simulink model "car"  (Simulink 8.0)
settings: Solver=ode15s  StartTime=0.0  StopTime=60  RelTol=1e-3
values from neighbouring files (symbols this model uses):
  i_f = r_back_sproket/r_front_sproket    (= 3.86486486486)    [meas_const.m]
  x = block.InputPort(1).Data    [parameterlookup.m]
undefined symbols (not defined in the file or in its folder): A_a, b, b_f, b_t, brake_gain, Bx, c_c, c_d, c_p, c_r, c_w, chaindrive, Cx, Dx, Ex, g, gearInertia, gearNumber, gearRatio, init_d, init_T, J_e, J_w, k, k_c, k_d, k_p, mass, N_idle, N_max, r_b, r_f, r_w, Rho_a, S, slope, T_max, tau_d, tau_e, x_dot
undefined symbols (not defined in the file): IdleControllerI, IdleControllerP, init_e, init_f, J_f, position
libraries: simulink x4
settings Model: Creator=erihe433  LastModifiedBy=johka546  ExtModeAutoUpdateStatusClock=off
settings DataIOCC: LimitDataPoints=off  SignalLoggingSaveFormat=ModelDataLogs  SaveOutput=off  SignalLogging=off  SignalLoggingName=sigsOut
settings OptimizationCC: InitFltsAndDblsToZero=on
settings DebuggingCC: SaveWithParameterizedLinksMsg=none  SignalResolutionControl=TryResolveAllWithWarning  SolverPrmCheckMsg=none  MultiTaskDSMMsg=warning  MultiTaskCondExecSysMsg=none  FcnCallInpInsideContextMsg=UseLocalSettings  StrictBusMsg=Warning
settings HardwareCC: TargetUnknown=on
settings RTWCC: IncludeERTFirstTime=on
settings GRTTargetCC: TargetFcnLib=ansi_tfl_tmw.mat  CombineOutputUpdateFcns=off  GRTInterface=on

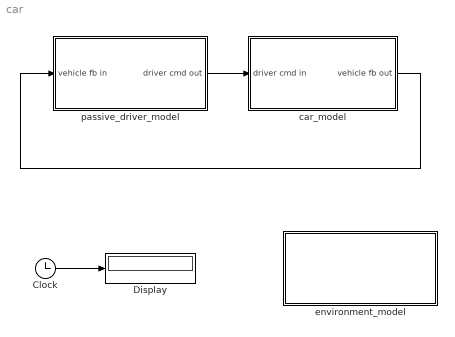
== system car ==
  Clock : Clock
  Display : Display
  car_model : Subsystem
  environment_model : Subsystem  AncestorBlock=capsim_lib/Environment/environment_model_jofr1  mask{Tamb=0, Pamb=0, pos=position, slope=slope}
      mask prompts: Tamb "Ambient Temperature [K]"; Pamb "Ambient Pressure [Pa]"; pos "positionvector in slope map [m]"; slope "slopevector in slope map [rad]"
      mask help: Environment settings
  passive_driver_model : Subsystem  AncestorBlock=capsim_lib/Driver/driver_model_template
      mask help: Driver model
  wires:
  car_model/1(vehicle fb out) -> passive_driver_model/1(vehicle fb in)
  passive_driver_model/1(driver cmd out) -> car_model/1(driver cmd in)
  Clock/1 -> Display/1

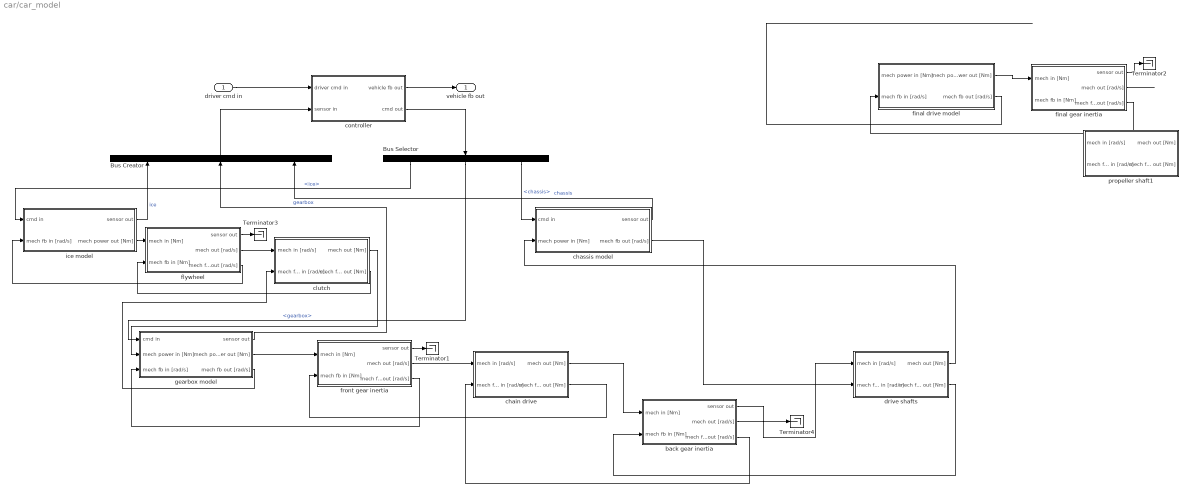
== system car/car_model ==
  driver cmd in : Inport
  Bus Creator : BusCreator  Inputs=3
  Bus Selector : BusSelector  OutputSignals=ice,gearbox,chassis
  Terminator{1..4} (4 alike) : Terminator
  back gear inertia : Subsystem  AncestorBlock=capsim_lib/Inertia/inertia_simple1_std  mask{mass=0, inertia=0, speedinit=init_f, angleinit=0}
      mask prompts: mass "Component mass [kg]"; inertia "Inertia [kg*m2]"; speedinit "Initial speed [rad/s]"; angleinit "Initial angle [rad]"
      mask help: Inertia
      mask Display: plot(-140,0,250,100,[40,40,80,80,40],[90,10,10,90,90],[80,40],[50,50],[80,40],[60,60],[80,40],[70,70],[80,40],[80,80],[80,40,40],[65,65,65],[80,40,40],[85,85,85],[80,40],[82,82],[80,40,40],[87,87,87],[80,40],[73,73],[80,40],[76,76],[80,40],[39,39],[80,40],[30,30],[80,40,40],[20,20,20],[80,40],[35,35],[80,40],[15,15],[80,40],[12,12],[80,40],[17,17],[80,40],[26,26],[80,40],[23,23],[40,10,10,40],[44,44,57,57])
  chain drive : Subsystem  AncestorBlock=capsim_lib/MechConverter/mechconverter_simple1_std  mask{mass=0, inertia=0, k_p=k_p, c_p=c_p}
      mask prompts: mass "Component mass [kg]"; inertia "Inertia [kg*m2]"; k_p "stiffness [Nm/rad]"; c_p "damping [Nms/rad]"
      mask help: Inertia
  chassis model : Subsystem  AncestorBlock=capsim_lib/Chassis/chassis_model_template
  clutch : Subsystem  AncestorBlock=capsim_lib/MechConverter/mechconverter_simple1_std  mask{mass=0, inertia=0, k_c=k_c, c_c=c_c}
      mask prompts: mass "Component mass [kg]"; inertia "Inertia [kg*m2]"; k_c "stiffness [Nm/rad]"; c_c "damping [Nms/rad]"
      mask help: Inertia
  controller : Subsystem  AncestorBlock=capsim_lib/Controller/controller_template
  drive shafts : Subsystem  AncestorBlock=capsim_lib/MechConverter/mechconverter_simple1_std  mask{mass=0, inertia=0, k_d=k_d, c_d=c_d}
      mask prompts: mass "Component mass [kg]"; inertia "Inertia [kg*m2]"; k_d "stiffness [Nm/rad]"; c_d "damping [Nms/rad]"
      mask help: Inertia
  final drive model : Subsystem  AncestorBlock=capsim_lib/Gearbox/gearbox_template
  final gear inertia : Subsystem  AncestorBlock=capsim_lib/Inertia/inertia_simple1_std  mask{mass=0, inertia=0, speedinit=init_f, angleinit=0}
      mask prompts: mass "Component mass [kg]"; inertia "Inertia [kg*m2]"; speedinit "Initial speed [rad/s]"; angleinit "Initial angle [rad]"
      mask help: Inertia
      mask Display: plot(-140,0,250,100,[40,40,80,80,40],[90,10,10,90,90],[80,40],[50,50],[80,40],[60,60],[80,40],[70,70],[80,40],[80,80],[80,40,40],[65,65,65],[80,40,40],[85,85,85],[80,40],[82,82],[80,40,40],[87,87,87],[80,40],[73,73],[80,40],[76,76],[80,40],[39,39],[80,40],[30,30],[80,40,40],[20,20,20],[80,40],[35,35],[80,40],[15,15],[80,40],[12,12],[80,40],[17,17],[80,40],[26,26],[80,40],[23,23],[40,10,10,40],[44,44,57,57])
  flywheel : Subsystem  AncestorBlock=capsim_lib/Inertia/inertia_simple1_std  mask{mass=0, inertia=0, speedinit=init_e, angleinit=0}
      mask prompts: mass "Component mass [kg]"; inertia "Inertia [kg*m2]"; speedinit "Initial speed [rad/s]"; angleinit "Initial angle [rad]"
      mask help: Inertia
      mask Display: plot(-140,0,250,100,[40,40,80,80,40],[90,10,10,90,90],[80,40],[50,50],[80,40],[60,60],[80,40],[70,70],[80,40],[80,80],[80,40,40],[65,65,65],[80,40,40],[85,85,85],[80,40],[82,82],[80,40,40],[87,87,87],[80,40],[73,73],[80,40],[76,76],[80,40],[39,39],[80,40],[30,30],[80,40,40],[20,20,20],[80,40],[35,35],[80,40],[15,15],[80,40],[12,12],[80,40],[17,17],[80,40],[26,26],[80,40],[23,23],[40,10,10,40],[44,44,57,57])
  front gear inertia : Subsystem  AncestorBlock=capsim_lib/Inertia/inertia_simple1_std  mask{mass=0, inertia=0, speedinit=init_f, angleinit=0}
      mask prompts: mass "Component mass [kg]"; inertia "Inertia [kg*m2]"; speedinit "Initial speed [rad/s]"; angleinit "Initial angle [rad]"
      mask help: Inertia
      mask Display: plot(-140,0,250,100,[40,40,80,80,40],[90,10,10,90,90],[80,40],[50,50],[80,40],[60,60],[80,40],[70,70],[80,40],[80,80],[80,40,40],[65,65,65],[80,40,40],[85,85,85],[80,40],[82,82],[80,40,40],[87,87,87],[80,40],[73,73],[80,40],[76,76],[80,40],[39,39],[80,40],[30,30],[80,40,40],[20,20,20],[80,40],[35,35],[80,40],[15,15],[80,40],[12,12],[80,40],[17,17],[80,40],[26,26],[80,40],[23,23],[40,10,10,40],[44,44,57,57])
  gearbox model : Subsystem  AncestorBlock=capsim_lib/Gearbox/gearbox_template
  ice model : Subsystem
  propeller shaft1 : Subsystem  AncestorBlock=capsim_lib/MechConverter/mechconverter_simple1_std  mask{mass=0, inertia=0, k_p=k_p, c_p=c_p}
      mask prompts: mass "Component mass [kg]"; inertia "Inertia [kg*m2]"; k_p "stiffness [Nm/rad]"; c_p "damping [Nms/rad]"
      mask help: Inertia
  vehicle fb out : Outport
  wires:
  controller/1(vehicle fb out) -> vehicle fb out/1
  driver cmd in/1 -> controller/1(driver cmd in)
  controller/2(cmd out) -> Bus Selector/1
  Bus Creator/1 -> controller/2(sensor in)
  Bus Selector/1 -> ice model/1(cmd in)  "<ice>"
  Bus Selector/3 -> chassis model/1(cmd in)  "<chassis>"
  chassis model/1(sensor out) -> Bus Creator/3  "chassis"
  ice model/2(mech power out [Nm]) -> flywheel/1(mech in [Nm])
  flywheel/3(mech fb out [rad/s]) -> ice model/2(mech fb in [rad/s])
  flywheel/2(mech out [rad/s]) -> clutch/1(mech in [rad/s])
  clutch/2(mech fb out [Nm]) -> flywheel/2(mech fb in [Nm])
  clutch/1(mech out [Nm]) -> gearbox model/2(mech power in [Nm])
  gearbox model/2(mech power out [Nm]) -> front gear inertia/1(mech in [Nm])
  gearbox model/3(mech fb out [rad/s]) -> clutch/2(mech fb in [rad/s])
  chain drive/2(mech fb out [Nm]) -> front gear inertia/2(mech fb in [Nm])
  chain drive/1(mech out [Nm]) -> back gear inertia/1(mech in [Nm])
  drive shafts/2(mech fb out [Nm]) -> back gear inertia/2(mech fb in [Nm])
  ? -> final drive model/1(mech power in [Nm])
  final drive model/2(mech fb out [rad/s]) -> ?
  final drive model/1(mech power out [Nm]) -> final gear inertia/1(mech in [Nm])
  final gear inertia/2(mech out [rad/s]) -> ?
  final gear inertia/3(mech fb out [rad/s]) -> final drive model/2(mech fb in [rad/s])
  drive shafts/1(mech out [Nm]) -> chassis model/2(mech power in [Nm])
  ? -> final gear inertia/2(mech fb in [Nm])
  chassis model/2(mech fb out [rad/s]) -> drive shafts/2(mech fb in [rad/s])
  ice model/1(sensor out) -> Bus Creator/1  "ice"
  flywheel/1(sensor out) -> Terminator3/1
  gearbox model/1(sensor out) -> Bus Creator/2  "gearbox"
  final gear inertia/1(sensor out) -> Terminator2/1
  Bus Selector/2 -> gearbox model/1(cmd in)  "<gearbox>"
  front gear inertia/2(mech out [rad/s]) -> chain drive/1(mech in [rad/s])
  front gear inertia/3(mech fb out [rad/s]) -> gearbox model/3(mech fb in [rad/s])
  front gear inertia/1(sensor out) -> Terminator1/1
  back gear inertia/3(mech fb out [rad/s]) -> chain drive/2(mech fb in [rad/s])
  back gear inertia/2(mech out [rad/s]) -> drive shafts/1(mech in [rad/s])
  back gear inertia/1(sensor out) -> Terminator4/1

== system car/environment_model ==
  Compare To Constant : simulink/Logic and Bit Operations/Compare To Constant  relop=<  const=1  OutDataTypeStr=uint8  ZeroCross=off
  Compare To Constant1 : simulink/Logic and Bit Operations/Compare To Constant  relop=<  const=1  OutDataTypeStr=uint8  ZeroCross=off
  Constant2 : Constant  Value=pos(end)
  Integrator : Integrator
  Logical Operator : Logic  Operator=OR  Inputs=3  AllPortsSameDT=off  OutDataTypeStr=boolean
  Relational Operator : RelationalOperator
  Stop Simulation1 : Stop
  To Workspace2 : ToWorkspace  VariableName=environmentout  SampleTime=-1
  slope as function of the distance : Lookup  InputValues=pos  Table=slope  LookUpMeth=Interpolation-Use End Values  SaturateOnIntegerOverflow=on
  tag scope: slope=global
  wires:
  [speed] -> Integrator/1, Compare To Constant/1
  Integrator/1 -> slope as function of the distance/1, Relational Operator/1  "distance"
  slope as function of the distance/1 -> [slope], To Workspace2/1
  Constant2/1 -> Relational Operator/2
  Logical Operator/1 -> Stop Simulation1/1
  Relational Operator/1 -> Logical Operator/1
  Compare To Constant/1 -> Logical Operator/2
  [wheelspeed] -> Compare To Constant1/1
  Compare To Constant1/1 -> Logical Operator/3

== system car/passive_driver_model ==
  vehicle fb in : Inport
  Bus Creator : BusCreator  Inputs=1
  Bus Selector : BusSelector  OutputSignals=velocity [m/s]
  From Workspace2 : FromWorkspace  VariableName=[InputT InputU]  SampleTime=0
  Terminator : Terminator
  driver cmd out : Outport
  wires:
  vehicle fb in/1 -> Bus Selector/1
  Bus Creator/1 -> driver cmd out/1
  Bus Selector/1 -> Terminator/1  "<velocity [m/s]>"
  From Workspace2/1 -> Bus Creator/1  "Torque demand [%]"

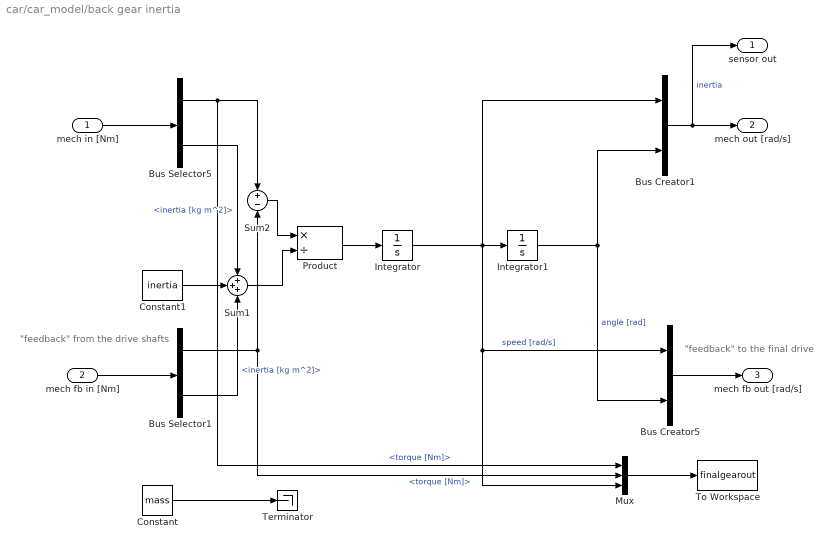
== system car/car_model/back gear inertia ==
  note: "feedback" to
      | the final drive
  note: "feedback" from
      | the drive shafts
  mech in [Nm] : Inport
  mech fb in [Nm] : Inport  Port=2
  Bus Creator1 : BusCreator  Inputs=2
  Bus Creator5 : BusCreator  Inputs=2
  Bus Selector1 : BusSelector  OutputSignals=torque [Nm],inertia [kg m^2]
  Bus Selector5 : BusSelector  OutputSignals=torque [Nm],inertia [kg m^2]
  Constant : Constant  Value=mass
  Constant1 : Constant  Value=inertia
  Integrator : Integrator  InitialCondition=speedinit
  Integrator1 : Integrator  InitialCondition=angleinit
  Mux : Mux  Inputs=3
  Product : Product  Inputs=*/  SaturateOnIntegerOverflow=on  OutDataTypeStr=Inherit: Same as first input
  Sum1 : Sum  Inputs=+++  SaturateOnIntegerOverflow=on
  Sum2 : Sum  Inputs=+|-  SaturateOnIntegerOverflow=on
  Terminator : Terminator
  To Workspace : ToWorkspace  VariableName=finalgearout  SampleTime=-1
  sensor out : Outport
  mech out [rad/s] : Outport  Port=2
  mech fb out [rad/s] : Outport  Port=3
  wires:
  Constant1/1 -> Sum1/2
  Bus Selector1/2 -> Sum1/3  "<inertia [kg m^2]>"
  Bus Selector1/1 -> Sum2/2, Mux/2  "<torque [Nm]>"
  Bus Selector5/2 -> Sum1/1  "<inertia [kg m^2]>"
  Bus Selector5/1 -> Sum2/1, Mux/1  "<torque [Nm]>"
  Bus Creator1/1 -> sensor out/1, mech out [rad/s]/1  "inertia"
  Bus Creator5/1 -> mech fb out [rad/s]/1
  mech fb in [Nm]/1 -> Bus Selector1/1
  Constant/1 -> Terminator/1
  mech in [Nm]/1 -> Bus Selector5/1
  Integrator1/1 -> Bus Creator5/2, Bus Creator1/2  "angle [rad]"
  Integrator/1 -> Bus Creator1/1, Integrator1/1, Bus Creator5/1, Mux/3  "speed [rad/s]"
  Product/1 -> Integrator/1
  Sum1/1 -> Product/2
  Sum2/1 -> Product/1
  Mux/1 -> To Workspace/1

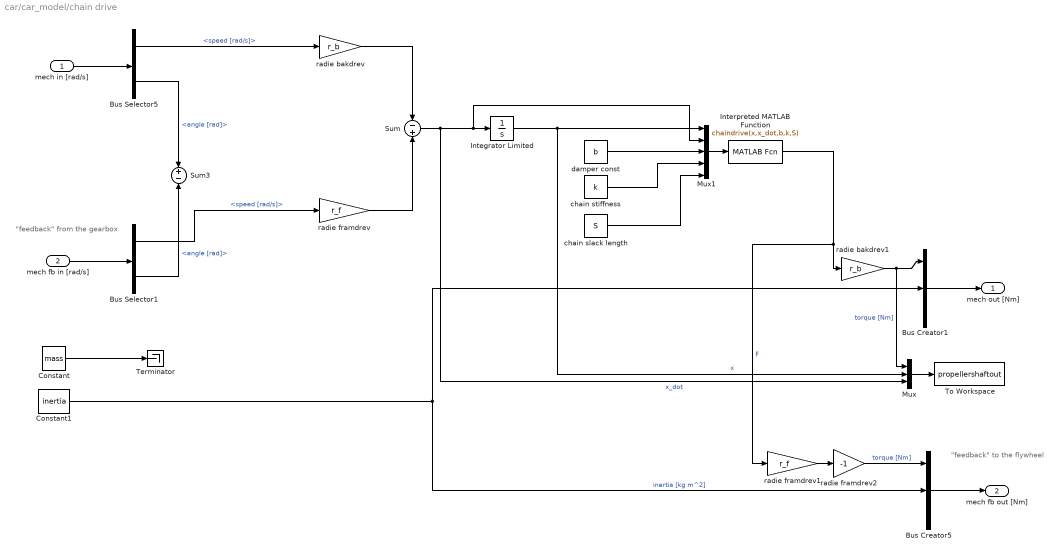
== system car/car_model/chain drive ==
  note: "feedback" to
      | the flywheel
  note: "feedback" from
      | the gearbox
  mech in [rad/s] : Inport
  mech fb in [rad/s] : Inport  Port=2
  " chain slack length" : Constant  Value=S
  Bus Creator1 : BusCreator  Inputs=3
  Bus Creator5 : BusCreator  Inputs=3
  Bus Selector1 : BusSelector  OutputSignals=speed [rad/s],angle [rad]
  Bus Selector5 : BusSelector  OutputSignals=speed [rad/s],angle [rad]
  Constant : Constant  Value=mass
  Constant1 : Constant  Value=inertia
  Integrator Limited : Integrator  LimitOutput=on  UpperSaturationLimit=S/2  LowerSaturationLimit=-S/2
  Interpreted MATLAB Function : MATLABFcn  MATLABFcn=chaindrive(x,x_dot,b,k,S)
  Mux : Mux  Inputs=3
  Mux1 : Mux  Inputs=5
  Sum : Sum  Inputs=-|+
  Sum3 : Sum  Inputs=+|-  SaturateOnIntegerOverflow=on
  Terminator : Terminator
  To Workspace : ToWorkspace  VariableName=propellershaftout  SampleTime=-1
  chain stiffness : Constant  Value=k
  damper const : Constant  Value=b
  radie bakdrev : Gain  Gain=r_b
  radie bakdrev1 : Gain  Gain=r_b
  radie framdrev : Gain  Gain=r_f
  radie framdrev1 : Gain  Gain=r_f
  radie framdrev2 : Gain  Gain=-1
  mech out [Nm] : Outport
  mech fb out [Nm] : Outport  Port=2
  wires:
  Constant1/1 -> Bus Creator5/2, Bus Creator1/2  "inertia [kg m^2]"
  Bus Selector1/2 -> Sum3/2  "<angle [rad]>"
  Bus Selector1/1 -> radie framdrev/1  "<speed [rad/s]>"
  Bus Selector5/2 -> Sum3/1  "<angle [rad]>"
  Bus Selector5/1 -> radie bakdrev/1  "<speed [rad/s]>"
  Bus Creator1/1 -> mech out [Nm]/1
  Bus Creator5/1 -> mech fb out [Nm]/1
  Constant/1 -> Terminator/1
  Mux/1 -> To Workspace/1
  mech fb in [rad/s]/1 -> Bus Selector1/1
  mech in [rad/s]/1 -> Bus Selector5/1
  Sum/1 -> Mux/3, Mux1/2, Integrator Limited/1  "x_dot"
  Integrator Limited/1 -> Mux/2, Mux1/1  "x"
  Mux1/1 -> Interpreted MATLAB Function/1
  damper const/1 -> Mux1/3
  chain stiffness/1 -> Mux1/4
  " chain slack length"/1 -> Mux1/5
  Interpreted MATLAB Function/1 -> radie bakdrev1/1, radie framdrev1/1  "F"
  radie bakdrev/1 -> Sum/1
  radie framdrev/1 -> Sum/2
  radie framdrev1/1 -> radie framdrev2/1
  radie framdrev2/1 -> Bus Creator5/1  "torque [Nm]"
  radie bakdrev1/1 -> Mux/1, Bus Creator1/1  "torque [Nm]"

== system car/car_model/chassis model ==
  cmd in : Inport
  mech power in [Nm] : Inport  Port=2
  chassis : Subsystem  mask{g=g, mass=mass, J_w=J_w, r_w=r_w, init_d=init_d, c_w=c_w, A_a=A_a, Rho_a=Rho_a, c_r=c_r, Bx=Bx, Cx=Cx, Dx=Dx, Ex=Ex}
      mask prompts: g "gravity constant [m/s^2]"; mass "vehicle mass [kg]"; J_w "wheel inertia [kg m^2]"; r_w "wheel radius [m]"; init_d "initial drive shaft speed [rad/s]"; c_w "air drag coefficient [-]"; A_a "max. vehicle cross section area [m^2]"; Rho_a "Air density [kg/m^3]"; c_r "rolling resistance coefficient [-]"; Bx "Magic Bx"; Cx "Magic Cx"; Dx "Magic Dx"; Ex "Magic Ex"
  local controller : Subsystem  mask{brake_gain=brake_gain}
      mask prompts: brake_gain "brake gain [Nm]"
  sensor out : Outport
  mech fb out [rad/s] : Outport  Port=2
  wires:
  local controller/2(ctrl out) -> chassis/1(ctrl in)
  cmd in/1 -> local controller/1(cmd in)
  local controller/1(sensor out) -> sensor out/1
  chassis/1(sensor out) -> local controller/2(sensor in)
  mech power in [Nm]/1 -> chassis/2(mech power in [Nm])
  chassis/2(mech fb out [rad/s]) -> mech fb out [rad/s]/1

== system car/car_model/clutch ==
  note: "feedback" from
      | the gearbox
  note: "feedback" to
      | the flywheel
  mech in [rad/s] : Inport
  mech fb in [rad/s] : Inport  Port=2
  Bus Creator1 : BusCreator  Inputs=2
  Bus Creator5 : BusCreator  Inputs=2
  Bus Selector1 : BusSelector  OutputSignals=speed [rad/s],angle [rad]
  Bus Selector5 : BusSelector  OutputSignals=speed [rad/s],angle [rad]
  Constant : Constant  Value=mass
  Constant1 : Constant  Value=inertia
  Gain : Gain  Gain=k_c
  Gain1 : Gain  Gain=c_c
  Mux : Mux  Inputs=3
  Sum2 : Sum  Inputs=+|-  SaturateOnIntegerOverflow=on
  Sum3 : Sum  Inputs=+|-  SaturateOnIntegerOverflow=on
  Sum4 : Sum
  Terminator : Terminator
  To Workspace : ToWorkspace  VariableName=clutchout  SampleTime=-1
  mech out [Nm] : Outport
  mech fb out [Nm] : Outport  Port=2
  wires:
  mech in [rad/s]/1 -> Bus Selector5/1
  mech fb in [rad/s]/1 -> Bus Selector1/1
  Mux/1 -> To Workspace/1
  Constant/1 -> Terminator/1
  Bus Creator5/1 -> mech fb out [Nm]/1
  Bus Creator1/1 -> mech out [Nm]/1
  Bus Selector5/1 -> Sum2/1  "<speed [rad/s]>"
  Bus Selector5/2 -> Sum3/1  "<angle [rad]>"
  Bus Selector1/1 -> Sum2/2  "<speed [rad/s]>"
  Bus Selector1/2 -> Sum3/2  "<angle [rad]>"
  Sum2/1 -> Gain1/1
  Sum3/1 -> Gain/1
  Gain1/1 -> Sum4/1, Mux/3
  Gain/1 -> Sum4/2, Mux/2
  Sum4/1 -> Bus Creator1/1, Bus Creator5/1, Mux/1  "torque [Nm]"
  Constant1/1 -> Bus Creator5/2, Bus Creator1/2  "inertia [kg m^2]"

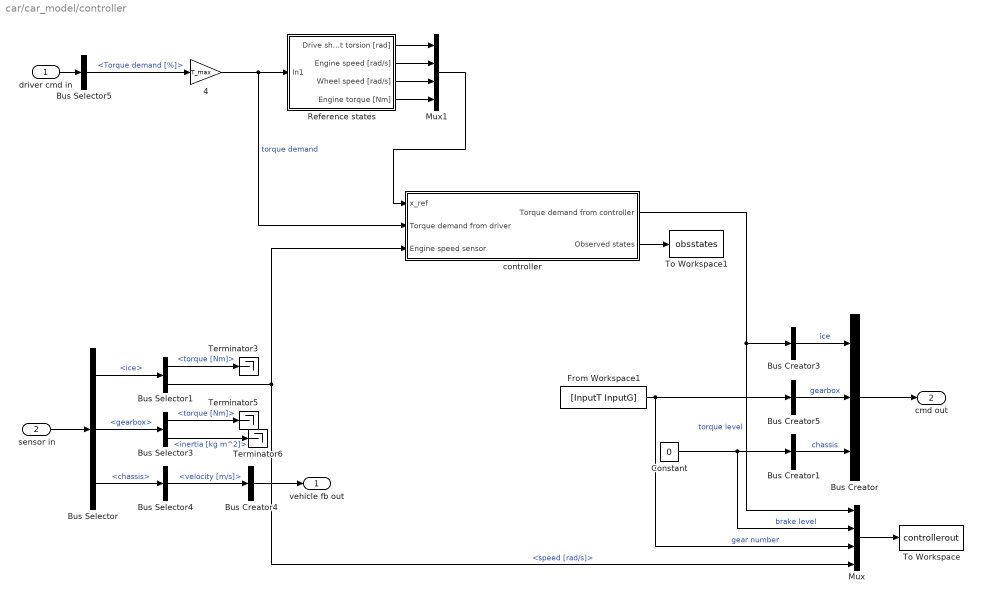
== system car/car_model/controller ==
  driver cmd in : Inport
  sensor in : Inport  Port=2
  4 : Gain  Gain=T_max
  Bus Creator : BusCreator  Inputs=3
  Bus Creator{1,3..5} (4 alike) : BusCreator  Inputs=1
  Bus Selector : BusSelector  OutputSignals=ice,gearbox,chassis
  Bus Selector1 : BusSelector  OutputSignals=torque [Nm],speed [rad/s]
  Bus Selector3 : BusSelector  OutputSignals=torque [Nm],inertia [kg m^2]
  Bus Selector4 : BusSelector  OutputSignals=velocity [m/s]
  Bus Selector5 : BusSelector  OutputSignals=Torque demand [%]
  Constant : Constant  Value=0
  From Workspace1 : FromWorkspace  VariableName=[InputT InputG]  SampleTime=0
  Mux : Mux
  Mux1 : Mux
  Reference states : Subsystem
  Terminator3 : Terminator
  Terminator5 : Terminator
  Terminator6 : Terminator
  To Workspace : ToWorkspace  VariableName=controllerout  SampleTime=-1
  To Workspace1 : ToWorkspace  VariableName=obsstates  SampleTime=-1
  controller : Subsystem
  vehicle fb out : Outport
  cmd out : Outport  Port=2
  wires:
  Bus Creator/1 -> cmd out/1
  Bus Creator3/1 -> Bus Creator/1  "ice"
  sensor in/1 -> Bus Selector/1
  Bus Selector/1 -> Bus Selector1/1  "<ice>"
  driver cmd in/1 -> Bus Selector5/1
  Bus Creator4/1 -> vehicle fb out/1
  Bus Selector5/1 -> 4/1  "<Torque demand [%]>"
  Bus Selector3/1 -> Terminator5/1  "<torque [Nm]>"
  Bus Selector3/2 -> Terminator6/1  "<inertia [kg m^2]>"
  Mux/1 -> To Workspace/1
  Bus Creator1/1 -> Bus Creator/3  "chassis"
  Bus Selector/2 -> Bus Selector3/1  "<gearbox>"
  Bus Selector/3 -> Bus Selector4/1  "<chassis>"
  Bus Selector1/1 -> Terminator3/1  "<torque [Nm]>"
  Bus Selector1/2 -> Mux/4, controller/3(Engine speed sensor)  "<speed [rad/s]>"
  Bus Selector4/1 -> Bus Creator4/1  "<velocity [m/s]>"
  Constant/1 -> Bus Creator1/1, Mux/2  "brake level"
  From Workspace1/1 -> Bus Creator5/1, Mux/3  "gear number"
  Bus Creator5/1 -> Bus Creator/2  "gearbox"
  4/1 -> Reference states/1(In1), controller/2(Torque demand from driver)  "torque demand"
  Reference states/1(Drive shaft torsion [rad]) -> Mux1/1
  Reference states/2(Engine speed [rad/s]) -> Mux1/2
  Reference states/3(Wheel speed [rad/s]) -> Mux1/3
  Reference states/4(Engine torque [Nm]) -> Mux1/4
  Mux1/1 -> controller/1(x_ref)
  controller/1(Torque demand from controller) -> Mux/1, Bus Creator3/1  "torque level"
  controller/2(Observed states) -> To Workspace1/1

== system car/car_model/drive shafts ==
  note: "feedback" from
      | the gearbox
  note: "feedback" to
      | the flywheel
  mech in [rad/s] : Inport
  mech fb in [rad/s] : Inport  Port=2
  Bus Creator1 : BusCreator  Inputs=2
  Bus Creator5 : BusCreator  Inputs=2
  Bus Selector1 : BusSelector  OutputSignals=speed [rad/s],angle [rad]
  Bus Selector5 : BusSelector  OutputSignals=speed [rad/s],angle [rad]
  Constant : Constant  Value=mass
  Constant1 : Constant  Value=inertia
  Gain : Gain  Gain=k_d
  Gain1 : Gain  Gain=c_d
  Mux : Mux  Inputs=3
  Sum2 : Sum  Inputs=+|-  SaturateOnIntegerOverflow=on
  Sum3 : Sum  Inputs=+|-  SaturateOnIntegerOverflow=on
  Sum4 : Sum
  Terminator : Terminator
  To Workspace : ToWorkspace  VariableName=driveshaftsout  SampleTime=-1
  mech out [Nm] : Outport
  mech fb out [Nm] : Outport  Port=2
  wires:
  mech in [rad/s]/1 -> Bus Selector5/1
  mech fb in [rad/s]/1 -> Bus Selector1/1
  Mux/1 -> To Workspace/1
  Constant/1 -> Terminator/1
  Bus Creator5/1 -> mech fb out [Nm]/1
  Bus Creator1/1 -> mech out [Nm]/1
  Bus Selector5/1 -> Sum2/1  "<speed [rad/s]>"
  Bus Selector5/2 -> Sum3/1  "<angle [rad]>"
  Bus Selector1/1 -> Sum2/2  "<speed [rad/s]>"
  Bus Selector1/2 -> Sum3/2  "<angle [rad]>"
  Sum2/1 -> Gain1/1, Mux/3
  Sum3/1 -> Gain/1, Mux/2
  Gain1/1 -> Sum4/1
  Gain/1 -> Sum4/2
  Sum4/1 -> Bus Creator1/1, Bus Creator5/1, Mux/1  "torque [Nm]"
  Constant1/1 -> Bus Creator5/2, Bus Creator1/2  "inertia [kg m^2]"

== system car/car_model/final drive model ==
  mech power in [Nm] : Inport
  mech fb in [rad/s] : Inport  Port=2
  final_drive : Subsystem  mask{mass=0, inertia=J_f, b_f=b_f, i_f=i_f}
      mask prompts: mass "mass [kg]"; inertia "inertia [kg m^2]"; b_f "Damping [Nm s/rad]"; i_f "Ratio [-]"
  mech power out [Nm] : Outport
  mech fb out [rad/s] : Outport  Port=2
  wires:
  mech fb in [rad/s]/1 -> final_drive/2(mech fb in [rad/s])
  final_drive/1(mech power out [Nm]) -> mech power out [Nm]/1
  mech power in [Nm]/1 -> final_drive/1(mech power in [Nm])
  final_drive/2(mech fb out [rad/s]) -> mech fb out [rad/s]/1

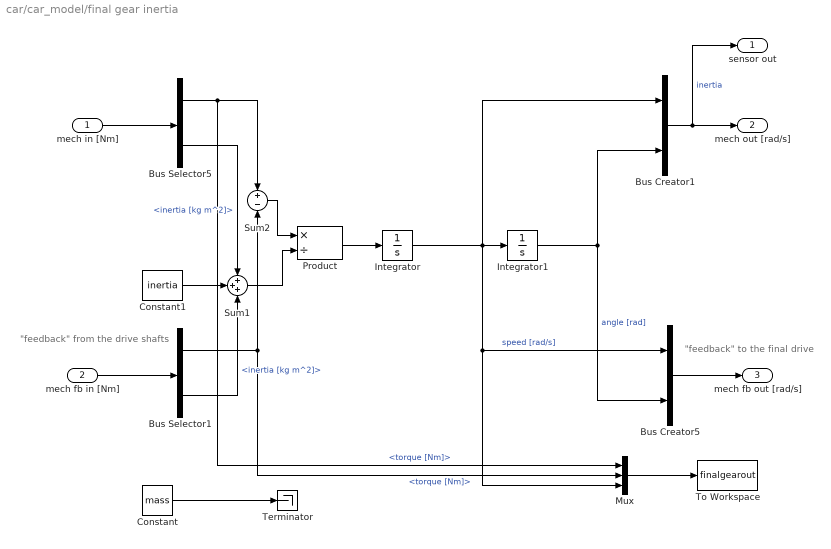
== system car/car_model/final gear inertia ==
  note: "feedback" to
      | the final drive
  note: "feedback" from
      | the drive shafts
  mech in [Nm] : Inport
  mech fb in [Nm] : Inport  Port=2
  Bus Creator1 : BusCreator  Inputs=2
  Bus Creator5 : BusCreator  Inputs=2
  Bus Selector1 : BusSelector  OutputSignals=torque [Nm],inertia [kg m^2]
  Bus Selector5 : BusSelector  OutputSignals=torque [Nm],inertia [kg m^2]
  Constant : Constant  Value=mass
  Constant1 : Constant  Value=inertia
  Integrator : Integrator  InitialCondition=speedinit
  Integrator1 : Integrator  InitialCondition=angleinit
  Mux : Mux  Inputs=3
  Product : Product  Inputs=*/  SaturateOnIntegerOverflow=on  OutDataTypeStr=Inherit: Same as first input
  Sum1 : Sum  Inputs=+++  SaturateOnIntegerOverflow=on
  Sum2 : Sum  Inputs=+|-  SaturateOnIntegerOverflow=on
  Terminator : Terminator
  To Workspace : ToWorkspace  VariableName=finalgearout  SampleTime=-1
  sensor out : Outport
  mech out [rad/s] : Outport  Port=2
  mech fb out [rad/s] : Outport  Port=3
  wires:
  Constant1/1 -> Sum1/2
  Bus Selector1/2 -> Sum1/3  "<inertia [kg m^2]>"
  Bus Selector1/1 -> Sum2/2, Mux/2  "<torque [Nm]>"
  Bus Selector5/2 -> Sum1/1  "<inertia [kg m^2]>"
  Bus Selector5/1 -> Sum2/1, Mux/1  "<torque [Nm]>"
  Bus Creator1/1 -> sensor out/1, mech out [rad/s]/1  "inertia"
  Bus Creator5/1 -> mech fb out [rad/s]/1
  mech fb in [Nm]/1 -> Bus Selector1/1
  Constant/1 -> Terminator/1
  mech in [Nm]/1 -> Bus Selector5/1
  Integrator1/1 -> Bus Creator5/2, Bus Creator1/2  "angle [rad]"
  Integrator/1 -> Bus Creator1/1, Integrator1/1, Bus Creator5/1, Mux/3  "speed [rad/s]"
  Product/1 -> Integrator/1
  Sum1/1 -> Product/2
  Sum2/1 -> Product/1
  Mux/1 -> To Workspace/1

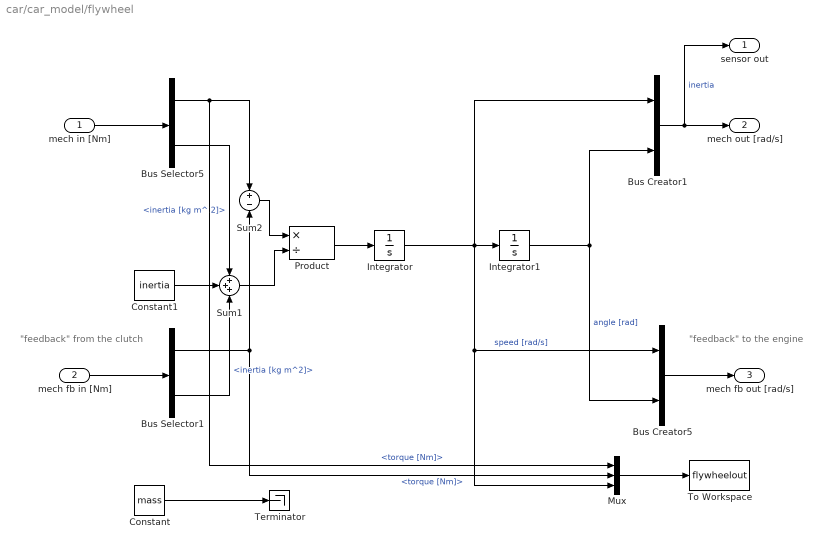
== system car/car_model/flywheel ==
  note: "feedback" to
      | the engine
  note: "feedback" from
      | the clutch
  mech in [Nm] : Inport
  mech fb in [Nm] : Inport  Port=2
  Bus Creator1 : BusCreator  Inputs=2
  Bus Creator5 : BusCreator  Inputs=2
  Bus Selector1 : BusSelector  OutputSignals=torque [Nm],inertia [kg m^2]
  Bus Selector5 : BusSelector  OutputSignals=torque [Nm],inertia [kg m^ 2]
  Constant : Constant  Value=mass
  Constant1 : Constant  Value=inertia
  Integrator : Integrator  InitialCondition=speedinit
  Integrator1 : Integrator  InitialCondition=angleinit
  Mux : Mux  Inputs=3
  Product : Product  Inputs=*/  SaturateOnIntegerOverflow=on  OutDataTypeStr=Inherit: Same as first input
  Sum1 : Sum  Inputs=+++  SaturateOnIntegerOverflow=on
  Sum2 : Sum  Inputs=+|-  SaturateOnIntegerOverflow=on
  Terminator : Terminator
  To Workspace : ToWorkspace  VariableName=flywheelout  SampleTime=-1
  sensor out : Outport
  mech out [rad/s] : Outport  Port=2
  mech fb out [rad/s] : Outport  Port=3
  wires:
  Mux/1 -> To Workspace/1
  Sum2/1 -> Product/1
  Sum1/1 -> Product/2
  Product/1 -> Integrator/1
  Integrator/1 -> Mux/3, Bus Creator5/1, Integrator1/1, Bus Creator1/1  "speed [rad/s]"
  Integrator1/1 -> Bus Creator5/2, Bus Creator1/2  "angle [rad]"
  mech in [Nm]/1 -> Bus Selector5/1
  Constant/1 -> Terminator/1
  mech fb in [Nm]/1 -> Bus Selector1/1
  Bus Creator5/1 -> mech fb out [rad/s]/1
  Bus Creator1/1 -> mech out [rad/s]/1, sensor out/1  "inertia"
  Bus Selector5/1 -> Mux/1, Sum2/1  "<torque [Nm]>"
  Bus Selector5/2 -> Sum1/1  "<inertia [kg m^ 2]>"
  Bus Selector1/1 -> Mux/2, Sum2/2  "<torque [Nm]>"
  Bus Selector1/2 -> Sum1/3  "<inertia [kg m^2]>"
  Constant1/1 -> Sum1/2

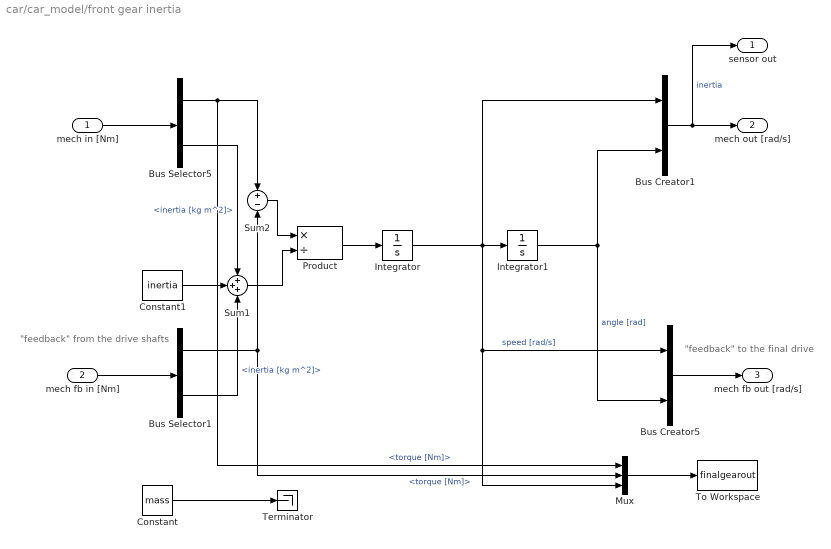
== system car/car_model/front gear inertia ==
  note: "feedback" from
      | the drive shafts
  note: "feedback" to
      | the final drive
  mech in [Nm] : Inport
  mech fb in [Nm] : Inport  Port=2
  Bus Creator1 : BusCreator  Inputs=2
  Bus Creator5 : BusCreator  Inputs=2
  Bus Selector1 : BusSelector  OutputSignals=torque [Nm],inertia [kg m^2]
  Bus Selector5 : BusSelector  OutputSignals=torque [Nm],inertia [kg m^2]
  Constant : Constant  Value=mass
  Constant1 : Constant  Value=inertia
  Integrator : Integrator  InitialCondition=speedinit
  Integrator1 : Integrator  InitialCondition=angleinit
  Mux : Mux  Inputs=3
  Product : Product  Inputs=*/  SaturateOnIntegerOverflow=on  OutDataTypeStr=Inherit: Same as first input
  Sum1 : Sum  Inputs=+++  SaturateOnIntegerOverflow=on
  Sum2 : Sum  Inputs=+|-  SaturateOnIntegerOverflow=on
  Terminator : Terminator
  To Workspace : ToWorkspace  VariableName=finalgearout  SampleTime=-1
  sensor out : Outport
  mech out [rad/s] : Outport  Port=2
  mech fb out [rad/s] : Outport  Port=3
  wires:
  Mux/1 -> To Workspace/1
  Sum2/1 -> Product/1
  Sum1/1 -> Product/2
  Product/1 -> Integrator/1
  Integrator/1 -> Mux/3, Bus Creator5/1, Integrator1/1, Bus Creator1/1  "speed [rad/s]"
  Integrator1/1 -> Bus Creator1/2, Bus Creator5/2  "angle [rad]"
  mech in [Nm]/1 -> Bus Selector5/1
  Constant/1 -> Terminator/1
  mech fb in [Nm]/1 -> Bus Selector1/1
  Bus Creator5/1 -> mech fb out [rad/s]/1
  Bus Creator1/1 -> mech out [rad/s]/1, sensor out/1  "inertia"
  Bus Selector5/1 -> Mux/1, Sum2/1  "<torque [Nm]>"
  Bus Selector5/2 -> Sum1/1  "<inertia [kg m^2]>"
  Bus Selector1/1 -> Mux/2, Sum2/2  "<torque [Nm]>"
  Bus Selector1/2 -> Sum1/3  "<inertia [kg m^2]>"
  Constant1/1 -> Sum1/2

== system car/car_model/gearbox model ==
  cmd in : Inport
  mech power in [Nm] : Inport  Port=2
  mech fb in [rad/s] : Inport  Port=3
  gearbox : Subsystem  mask{mass=0, inertia=0, b_t=b_t}
      mask prompts: mass "mass [kg]"; inertia "inertia [kg m^2]"; b_t "Damping [Nm s/rad]"
  local controller : Subsystem  mask{gearNumber=gearNumber, gearRatio=gearRatio, gearInertia=gearInertia}
      mask prompts: gearNumber "gear number vector"; gearRatio "gear ratio vector"; gearInertia "gear inertia vector"
  sensor out : Outport
  mech power out [Nm] : Outport  Port=2
  mech fb out [rad/s] : Outport  Port=3
  wires:
  gearbox/3(mech fb out [rad/s]) -> mech fb out [rad/s]/1
  mech power in [Nm]/1 -> gearbox/2(mech power in [Nm])
  gearbox/2(mech power out [Nm]) -> mech power out [Nm]/1
  mech fb in [rad/s]/1 -> gearbox/3(mech fb in [rad/s])
  gearbox/1(sensor out) -> local controller/2(sensor in)
  local controller/1(sensor out) -> sensor out/1
  cmd in/1 -> local controller/1(cmd in)
  local controller/2(ctrl) -> gearbox/1(ctrl)

== system car/car_model/ice model ==
  cmd in : Inport
  mech fb in [rad/s] : Inport  Port=2
  ice : Subsystem  mask{mass=0, inertia=J_e, tau_d=tau_d, tau_e=tau_e, init_T=init_T}
      mask prompts: mass "mass [kg]"; inertia "inertia [kg m^2]"; tau_d "time delay [s]"; tau_e "time constant [s]"; init_T "initial torque [Nm]"
  local controller : Subsystem  mask{T_max=T_max, N_max=N_max, N_idle=N_idle, P=IdleControllerP, I=IdleControllerI}
      mask prompts: T_max "maximum torque [Nm]"; N_max "maximum speed [rad/s]"; N_idle "Idle controller reference value [rad/s]"; P "Idle controller proportional gain"; I "Idle controller integral gain"
  sensor out : Outport
  mech power out [Nm] : Outport  Port=2
  wires:
  ice/2(mech power out [Nm]) -> mech power out [Nm]/1
  mech fb in [rad/s]/1 -> ice/2(mech fb in [rad/s])
  ice/1(sensor out) -> local controller/2(sensor in)
  local controller/1(sensor out) -> sensor out/1
  cmd in/1 -> local controller/1(cmd in)
  local controller/2(ctrl) -> ice/1(ctrl)

== system car/car_model/propeller shaft1 ==
  note: "feedback" from
      | the gearbox
  note: "feedback" to
      | the flywheel
  mech in [rad/s] : Inport
  mech fb in [rad/s] : Inport  Port=2
  Bus Creator1 : BusCreator  Inputs=2
  Bus Creator5 : BusCreator  Inputs=2
  Bus Selector1 : BusSelector  OutputSignals=speed [rad/s],angle [rad]
  Bus Selector5 : BusSelector  OutputSignals=speed [rad/s],angle [rad]
  Constant : Constant  Value=mass
  Constant1 : Constant  Value=inertia
  Gain : Gain  Gain=k_p
  Gain1 : Gain  Gain=c_p
  Mux : Mux  Inputs=3
  Sum2 : Sum  Inputs=+|-  SaturateOnIntegerOverflow=on
  Sum3 : Sum  Inputs=+|-  SaturateOnIntegerOverflow=on
  Sum4 : Sum
  Terminator : Terminator
  To Workspace : ToWorkspace  VariableName=propellershaftout  SampleTime=-1
  mech out [Nm] : Outport
  mech fb out [Nm] : Outport  Port=2
  wires:
  mech in [rad/s]/1 -> Bus Selector5/1
  mech fb in [rad/s]/1 -> Bus Selector1/1
  Mux/1 -> To Workspace/1
  Constant/1 -> Terminator/1
  Bus Creator5/1 -> mech fb out [Nm]/1
  Bus Creator1/1 -> mech out [Nm]/1
  Bus Selector5/1 -> Sum2/1  "<speed [rad/s]>"
  Bus Selector5/2 -> Sum3/1  "<angle [rad]>"
  Bus Selector1/1 -> Sum2/2  "<speed [rad/s]>"
  Bus Selector1/2 -> Sum3/2  "<angle [rad]>"
  Sum2/1 -> Gain1/1
  Sum3/1 -> Gain/1
  Gain1/1 -> Mux/3, Sum4/1
  Gain/1 -> Mux/2, Sum4/2
  Sum4/1 -> Bus Creator1/1, Bus Creator5/1, Mux/1  "torque [Nm]"
  Constant1/1 -> Bus Creator5/2, Bus Creator1/2  "inertia [kg m^2]"

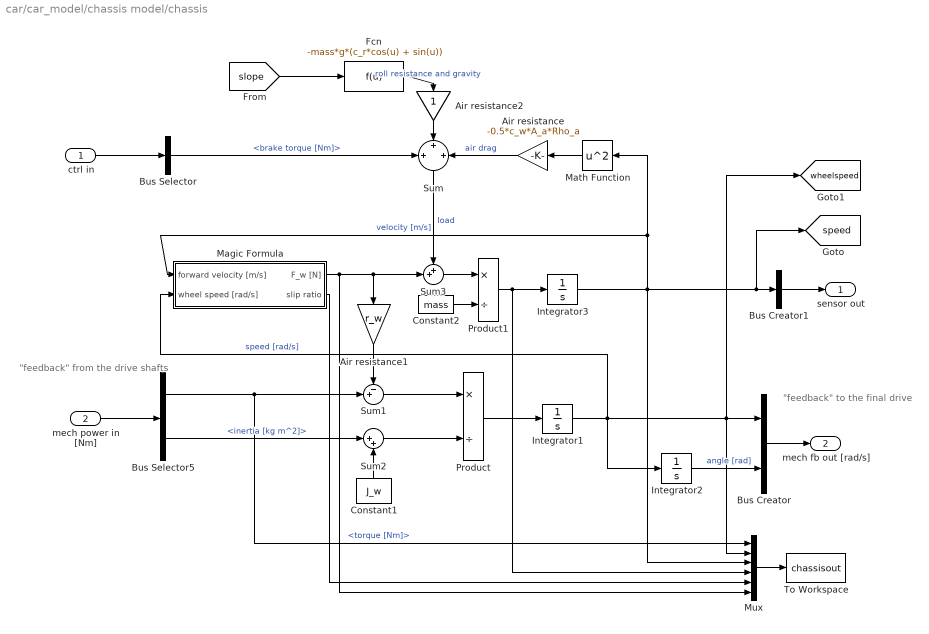
== system car/car_model/chassis model/chassis ==
  note: "feedback" from
      | the drive shafts
  note: "feedback" to
      | the final drive
  ctrl in : Inport
  mech power in [Nm] : Inport  Port=2
  Air resistance : Gain  Gain=-0.5*c_w*A_a*Rho_a  SaturateOnIntegerOverflow=on  OutDataTypeStr=Inherit: Same as input  ParamDataTypeStr=Inherit: Same as input
  Air resistance1 : Gain  Gain=r_w  SaturateOnIntegerOverflow=on  OutDataTypeStr=Inherit: Same as input  ParamDataTypeStr=Inherit: Same as input
  Air resistance2 : Gain  SaturateOnIntegerOverflow=on  OutDataTypeStr=Inherit: Same as input  ParamDataTypeStr=Inherit: Same as input
  Bus Creator : BusCreator  Inputs=2
  Bus Creator1 : BusCreator  Inputs=1
  Bus Selector : BusSelector  OutputSignals=brake torque [Nm]
  Bus Selector5 : BusSelector  OutputSignals=torque [Nm],inertia [kg m^2]
  Constant1 : Constant  Value=J_w
  Constant2 : Constant  Value=mass
  Fcn : Fcn  Expr=-mass*g*(c_r*cos(u) + sin(u))
  Integrator1 : Integrator  InitialCondition=init_d
  Integrator2 : Integrator
  Integrator3 : Integrator  InitialCondition=init_d*r_w
  Magic Formula : Subsystem
  Math Function : Math  Operator=square  SaturateOnIntegerOverflow=on
  Mux : Mux  Inputs=6
  Product : Product  Inputs=*/  SaturateOnIntegerOverflow=on  OutDataTypeStr=Inherit: Same as first input
  Product1 : Product  Inputs=*/  SaturateOnIntegerOverflow=on  OutDataTypeStr=Inherit: Same as first input
  Sum : Sum  Inputs=+|+|+  SaturateOnIntegerOverflow=on
  Sum1 : Sum  Inputs=-+|  SaturateOnIntegerOverflow=on
  Sum2 : Sum  Inputs=|++  SaturateOnIntegerOverflow=on
  Sum3 : Sum  Inputs=++|  SaturateOnIntegerOverflow=on
  To Workspace : ToWorkspace  VariableName=chassisout  SampleTime=-1
  sensor out : Outport
  mech fb out [rad/s] : Outport  Port=2
  tag scope: speed=global, wheelspeed=global
  wires:
  Mux/1 -> To Workspace/1
  Integrator2/1 -> Bus Creator/2  "angle [rad]"
  Bus Selector5/2 -> Sum2/1  "<inertia [kg m^2]>"
  Bus Selector5/1 -> Mux/1, Sum1/2  "<torque [Nm]>"
  mech power in [Nm]/1 -> Bus Selector5/1
  Bus Creator/1 -> mech fb out [rad/s]/1
  ctrl in/1 -> Bus Selector/1
  [slope] -> Fcn/1
  Math Function/1 -> Air resistance/1
  Integrator1/1 -> Integrator2/1, Magic Formula/2(wheel speed [rad/s]), Mux/2, Bus Creator/1, [wheelspeed]  "speed [rad/s]"
  Air resistance/1 -> Sum/3  "air drag"
  Fcn/1 -> Air resistance2/1  "roll resistance and gravity"
  Bus Selector/1 -> Sum/1  "<brake torque [Nm]>"
  Bus Creator1/1 -> sensor out/1
  Sum2/1 -> Product/2
  Sum1/1 -> Product/1
  Product/1 -> Integrator1/1
  Constant1/1 -> Sum2/2
  Sum/1 -> Sum3/1  "load"
  Magic Formula/1(F_w [N]) -> Sum3/2, Air resistance1/1, Mux/6
  Sum3/1 -> Product1/1
  Constant2/1 -> Product1/2
  Product1/1 -> Integrator3/1, Mux/4
  Integrator3/1 -> Mux/3, Math Function/1, Magic Formula/1(forward velocity [m/s]), Bus Creator1/1, [speed]  "velocity [m/s]"
  Air resistance1/1 -> Sum1/1
  Magic Formula/2(slip ratio) -> Mux/5
  Air resistance2/1 -> Sum/2

== system car/car_model/chassis model/local controller ==
  cmd in : Inport
  sensor in : Inport  Port=2
  Bus Creator : BusCreator  Inputs=1
  Bus Selector : BusSelector  OutputSignals=brake level
  Saturation : Saturate  UpperLimit=1  LowerLimit=0
  brake_gain : Gain  Gain=-brake_gain  SaturateOnIntegerOverflow=on  OutDataTypeStr=Inherit: Same as input  ParamDataTypeStr=Inherit: Same as input
  sensor out : Outport
  ctrl out : Outport  Port=2
  wires:
  cmd in/1 -> Bus Selector/1
  Bus Selector/1 -> Saturation/1  "<brake level>"
  Saturation/1 -> brake_gain/1
  brake_gain/1 -> Bus Creator/1  "brake torque [Nm]"
  Bus Creator/1 -> ctrl out/1
  sensor in/1 -> sensor out/1

== system car/car_model/controller/Reference states ==
  In1 : Inport
  1 : Gain  Gain=i_f*gearRatio(1)
  2 : Gain  Gain=1/tau_e
  5 : Gain  Gain=1/r_w
  6 : Gain  Gain=i_f*gearRatio(1)/k_d
  Add : Sum  Inputs=+-
  Fcn : Fcn  Expr=(i_f*gearRatio(1)/r_w*u(1)-0.5*Rho_a*c_w*A_a*u(2)^2-mass*g*c_r)/(mass+i_f^2*gearRatio(1)^2/r_w^2*J_e)
  Integrator : Integrator  InitialCondition=28/3.6
  Integrator1 : Integrator  InitialCondition=-8
  Mux6 : Mux  Inputs=2
  Drive shaft torsion [rad] : Outport
  Engine speed [rad/s] : Outport  Port=2
  Wheel speed [rad/s] : Outport  Port=3
  Engine torque [Nm] : Outport  Port=4
  wires:
  Fcn/1 -> Integrator/1
  Integrator/1 -> Mux6/2, 5/1  "v"
  Mux6/1 -> Fcn/1
  5/1 -> Wheel speed [rad/s]/1, 1/1
  6/1 -> Drive shaft torsion [rad]/1
  1/1 -> Engine speed [rad/s]/1
  Integrator1/1 -> Mux6/1, Engine torque [Nm]/1, 6/1, Add/2
  In1/1 -> Add/1
  Add/1 -> 2/1
  2/1 -> Integrator1/1

== system car/car_model/controller/controller ==
  note: Construct an observer for the vehicle using the engine speed sensor.
      | Then use the given reference states (x_ref) and design a state feedback controller to damp the driveline oscillations.
  note: Connect your observed states
      | hear to plot them in Figure 3
  x_ref : Inport
  Torque demand from driver : Inport  Port=2
  Engine speed sensor : Inport  Port=3
  Ground : Ground
  Ground1 : Ground
  Manual Switch : ManualSwitch
  Mux : Mux
  Terminator1 : Terminator
  Terminator3 : Terminator
  Torque demand from controller : Outport
  Observed states : Outport  Port=2
  wires:
  Torque demand from driver/1 -> Manual Switch/1
  Manual Switch/1 -> Torque demand from controller/1
  Engine speed sensor/1 -> Terminator3/1
  x_ref/1 -> Terminator1/1
  Ground/1 -> Manual Switch/2
  Ground1/1 -> Mux/1, Mux/2, Mux/3, Mux/4
  Mux/1 -> Observed states/1

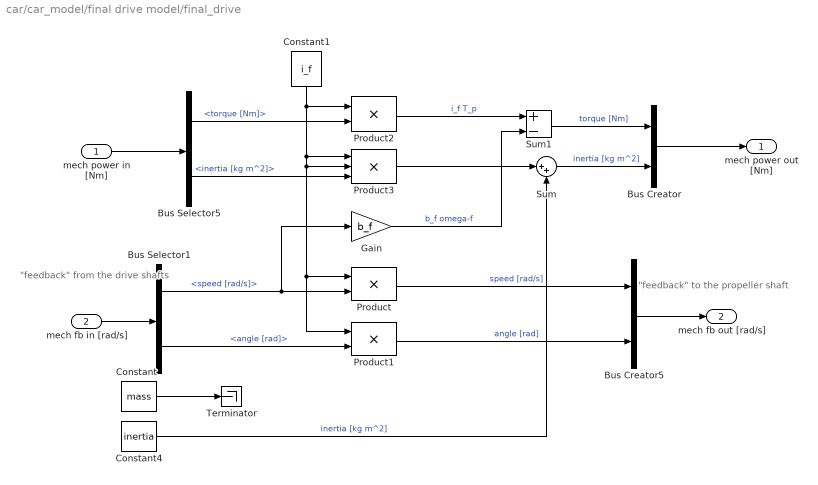
== system car/car_model/final drive model/final_drive ==
  note: "feedback" to
      | the propeller shaft
  note: "feedback" from
      | the drive shafts
  mech power in [Nm] : Inport
  mech fb in [rad/s] : Inport  Port=2
  Bus Creator : BusCreator  Inputs=2
  Bus Creator5 : BusCreator  Inputs=2
  Bus Selector1 : BusSelector  OutputSignals=speed [rad/s],angle [rad]
  Bus Selector5 : BusSelector  OutputSignals=torque [Nm],inertia [kg m^2]
  Constant : Constant  Value=mass
  Constant1 : Constant  Value=i_f
  Constant4 : Constant  Value=inertia
  Gain : Gain  Gain=b_f
  Product : Product  Inputs=**  SaturateOnIntegerOverflow=on  OutDataTypeStr=Inherit: Same as first input
  Product1 : Product  Inputs=**  SaturateOnIntegerOverflow=on  OutDataTypeStr=Inherit: Same as first input
  Product2 : Product  SaturateOnIntegerOverflow=on  OutDataTypeStr=Inherit: Same as first input
  Product3 : Product  Inputs=3  SaturateOnIntegerOverflow=on  OutDataTypeStr=Inherit: Same as first input
  Sum : Sum  Inputs=|++
  Sum1 : Sum  Inputs=+-
  Terminator : Terminator
  mech power out [Nm] : Outport
  mech fb out [rad/s] : Outport  Port=2
  wires:
  Gain/1 -> Sum1/2  "b_f omega-f"
  Sum1/1 -> Bus Creator/1  "torque [Nm]"
  Product2/1 -> Sum1/1  "i_f T_p"
  Sum/1 -> Bus Creator/2  "inertia [kg m^2]"
  Product3/1 -> Sum/1
  Constant4/1 -> Sum/2  "inertia [kg m^2]"
  Constant1/1 -> Product1/1, Product/1, Product3/2, Product3/1, Product2/1
  mech fb in [rad/s]/1 -> Bus Selector1/1
  Bus Creator/1 -> mech power out [Nm]/1
  Bus Selector1/2 -> Product1/2  "<angle [rad]>"
  Constant/1 -> Terminator/1
  Bus Selector1/1 -> Gain/1, Product/2  "<speed [rad/s]>"
  mech power in [Nm]/1 -> Bus Selector5/1
  Bus Selector5/1 -> Product2/2  "<torque [Nm]>"
  Bus Selector5/2 -> Product3/3  "<inertia [kg m^2]>"
  Product/1 -> Bus Creator5/1  "speed [rad/s]"
  Product1/1 -> Bus Creator5/2  "angle [rad]"
  Bus Creator5/1 -> mech fb out [rad/s]/1

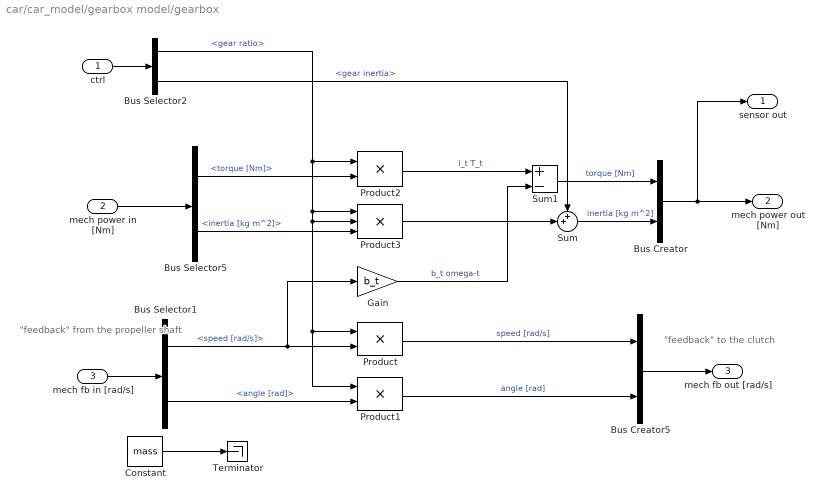
== system car/car_model/gearbox model/gearbox ==
  note: "feedback" from
      | the propeller shaft
  note: "feedback" to
      | the clutch
  ctrl : Inport
  mech power in [Nm] : Inport  Port=2
  mech fb in [rad/s] : Inport  Port=3
  Bus Creator : BusCreator  Inputs=2
  Bus Creator5 : BusCreator  Inputs=2
  Bus Selector1 : BusSelector  OutputSignals=speed [rad/s],angle [rad]
  Bus Selector2 : BusSelector  OutputSignals=gear ratio,gear inertia
  Bus Selector5 : BusSelector  OutputSignals=torque [Nm],inertia [kg m^2]
  Constant : Constant  Value=mass
  Gain : Gain  Gain=b_t
  Product : Product  Inputs=**  SaturateOnIntegerOverflow=on  OutDataTypeStr=Inherit: Same as first input
  Product1 : Product  Inputs=**  SaturateOnIntegerOverflow=on  OutDataTypeStr=Inherit: Same as first input
  Product2 : Product  SaturateOnIntegerOverflow=on  OutDataTypeStr=Inherit: Same as first input
  Product3 : Product  Inputs=3  SaturateOnIntegerOverflow=on  OutDataTypeStr=Inherit: Same as first input
  Sum : Sum  Inputs=++|
  Sum1 : Sum  Inputs=+-
  Terminator : Terminator
  sensor out : Outport
  mech power out [Nm] : Outport  Port=2
  mech fb out [rad/s] : Outport  Port=3
  wires:
  Bus Creator5/1 -> mech fb out [rad/s]/1
  Product1/1 -> Bus Creator5/2  "angle [rad]"
  Product/1 -> Bus Creator5/1  "speed [rad/s]"
  Bus Selector5/2 -> Product3/3  "<inertia [kg m^2]>"
  Bus Selector5/1 -> Product2/2  "<torque [Nm]>"
  mech power in [Nm]/1 -> Bus Selector5/1
  Bus Selector1/1 -> Product/2, Gain/1  "<speed [rad/s]>"
  Constant/1 -> Terminator/1
  Bus Selector1/2 -> Product1/2  "<angle [rad]>"
  Bus Creator/1 -> mech power out [Nm]/1, sensor out/1
  mech fb in [rad/s]/1 -> Bus Selector1/1
  ctrl/1 -> Bus Selector2/1
  Bus Selector2/1 -> Product/1, Product1/1, Product3/2, Product3/1, Product2/1  "<gear ratio>"
  Product2/1 -> Sum1/1  "i_t T_t"
  Sum1/1 -> Bus Creator/1  "torque [Nm]"
  Gain/1 -> Sum1/2  "b_t omega-t"
  Bus Selector2/2 -> Sum/1  "<gear inertia>"
  Sum/1 -> Bus Creator/2  "inertia [kg m^2]"
  Product3/1 -> Sum/2

== system car/car_model/gearbox model/local controller ==
  cmd in : Inport
  sensor in : Inport  Port=2
  Bus Creator : BusCreator  Inputs=2
  Bus Selector : BusSelector  OutputSignals=gear number
  gear number to inertia table : Lookup  InputValues=gearNumber  Table=gearInertia  LookUpMeth=Interpolation-Use End Values  SaturateOnIntegerOverflow=on
  gear number to ratio table : Lookup  InputValues=gearNumber  Table=gearRatio  LookUpMeth=Interpolation-Use End Values  SaturateOnIntegerOverflow=on
  sensor out : Outport
  ctrl : Outport  Port=2
  wires:
  sensor in/1 -> sensor out/1
  cmd in/1 -> Bus Selector/1
  Bus Selector/1 -> gear number to ratio table/1, gear number to inertia table/1  "<gear number>"
  Bus Creator/1 -> ctrl/1
  gear number to ratio table/1 -> Bus Creator/1  "gear ratio"
  gear number to inertia table/1 -> Bus Creator/2  "gear inertia"

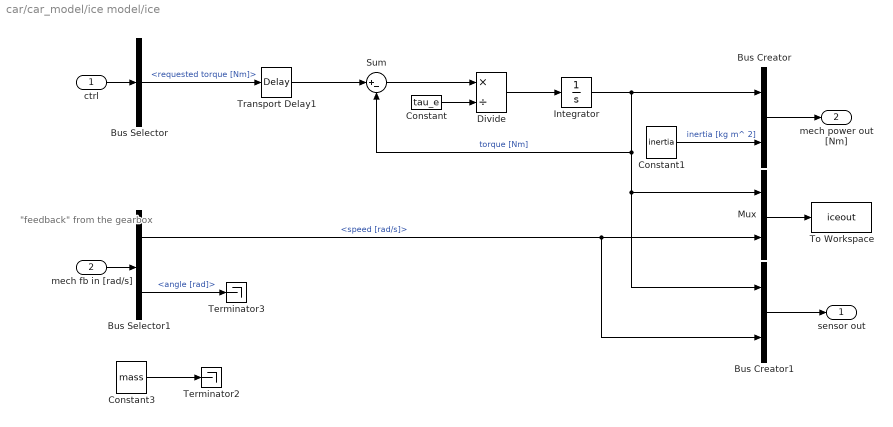
== system car/car_model/ice model/ice ==
  note: "feedback" from
      | the gearbox
  ctrl : Inport
  mech fb in [rad/s] : Inport  Port=2
  Bus Creator : BusCreator  Inputs=2
  Bus Creator1 : BusCreator  Inputs=2
  Bus Selector : BusSelector  OutputSignals=requested torque [Nm]
  Bus Selector1 : BusSelector  OutputSignals=speed [rad/s],angle [rad]
  Constant : Constant  Value=tau_e
  Constant1 : Constant  Value=inertia
  Constant3 : Constant  Value=mass
  Divide : Product  Inputs=*/
  Integrator : Integrator  InitialCondition=init_T
  Mux : Mux  Inputs=2
  Sum : Sum  Inputs=|+-
  Terminator2 : Terminator
  Terminator3 : Terminator
  To Workspace : ToWorkspace  VariableName=iceout  SampleTime=-1
  Transport Delay1 : TransportDelay  DelayTime=tau_d
  sensor out : Outport
  mech power out [Nm] : Outport  Port=2
  wires:
  Constant3/1 -> Terminator2/1
  Bus Creator1/1 -> sensor out/1
  Mux/1 -> To Workspace/1
  Bus Selector1/2 -> Terminator3/1  "<angle [rad]>"
  Bus Creator/1 -> mech power out [Nm]/1
  mech fb in [rad/s]/1 -> Bus Selector1/1
  ctrl/1 -> Bus Selector/1
  Constant/1 -> Divide/2
  Divide/1 -> Integrator/1
  Sum/1 -> Divide/1
  Integrator/1 -> Bus Creator/1, Sum/2, Mux/1, Bus Creator1/1  "torque [Nm]"
  Constant1/1 -> Bus Creator/2  "inertia [kg m^ 2]"
  Bus Selector1/1 -> Mux/2, Bus Creator1/2  "<speed [rad/s]>"
  Bus Selector/1 -> Transport Delay1/1  "<requested torque [Nm]>"
  Transport Delay1/1 -> Sum/1

== system car/car_model/ice model/local controller ==
  cmd in : Inport
  sensor in : Inport  Port=2
  Bus Creator : BusCreator  Inputs=1
  Bus Selector : BusSelector  OutputSignals=torque level
  Bus Selector1 : BusSelector  OutputSignals=speed [rad/s]
  Compare To Constant : simulink/Logic and Bit Operations/Compare To Constant  relop=>=  const=N_max*0.99  OutDataTypeStr=uint8  ZeroCross=off
  Compare To Constant1 : simulink/Logic and Bit Operations/Compare To Constant  relop=<=  const=N_idle*1.15  OutDataTypeStr=uint8  ZeroCross=off
  Idle controller : Subsystem
  Max speed controller : Subsystem
  MinMax : MinMax  Function=max  Inputs=2
  MinMax1 : MinMax  Inputs=2
  Saturation : Saturate  UpperLimit=T_max  LowerLimit=-T_max
  gain : Gain  SaturateOnIntegerOverflow=on  OutDataTypeStr=Inherit: Same as input  ParamDataTypeStr=Inherit: Same as input
  sensor out : Outport
  ctrl : Outport  Port=2
  wires:
  Max speed controller/1(req_T) -> MinMax1/2
  Compare To Constant/1 -> Max speed controller/Enable
  MinMax/1 -> Bus Creator/1  "requested torque [Nm]"
  [DriverRequstedTorque] -> Idle controller/2(Driver request)
  Compare To Constant1/1 -> Idle controller/Enable
  Idle controller/1(req_T) -> MinMax/2
  Bus Selector1/1 -> Compare To Constant/1, Compare To Constant1/1, Idle controller/1(w_e)  "<speed [rad/s]>"
  gain/1 -> MinMax1/1, [DriverRequstedTorque]
  MinMax1/1 -> MinMax/1
  sensor in/1 -> sensor out/1, Bus Selector1/1
  Bus Creator/1 -> ctrl/1
  Saturation/1 -> gain/1
  Bus Selector/1 -> Saturation/1  "<torque level>"
  cmd in/1 -> Bus Selector/1

== system car/car_model/chassis model/chassis/Magic Formula ==
  note: Note: The SAE definition of the slip ratio kappa is used.
  forward velocity [m/s] : Inport
  wheel speed [rad/s] : Inport  Port=2
  Constant : Constant
  Divide : Product  Inputs=*/
  Gain : Gain  Gain=r_w
  Magic Formula : Fcn  Expr=Dx*sin(Cx*atan(Bx*u-Ex*(Bx*u-atan(Bx*u))))
  Sum3 : Sum  Inputs=-+|
  F_w [N] : Outport
  slip ratio : Outport  Port=2
  wires:
  Gain/1 -> Divide/1
  Sum3/1 -> Magic Formula/1, slip ratio/1  "kappa"
  Constant/1 -> Sum3/1
  Divide/1 -> Sum3/2
  wheel speed [rad/s]/1 -> Gain/1
  Magic Formula/1 -> F_w [N]/1
  forward velocity [m/s]/1 -> Divide/2

== system car/car_model/ice model/local controller/Idle controller ==
  w_e : Inport
  Driver request : Inport  Port=2
  Enable : EnablePort  StatesWhenEnabling=reset  PropagateVarSize=During execution
  Constant : Constant  Value=N_idle
  Gain : Gain  Gain=P
  Gain1 : Gain  Gain=I
  Integrator : Integrator  InitialConditionSource=external
  Sum : Sum  Inputs=+|+
  Sum1 : Sum  Inputs=|-+
  Sum2 : Sum  Inputs=-+|
  req_T : Outport  OutputWhenDisabled=reset  InitialOutput=-T_max
  wires:
  Sum2/1 -> Integrator/2
  Driver request/1 -> Sum2/2
  Constant/1 -> Sum1/2
  Sum1/1 -> Gain1/1, Gain/1
  w_e/1 -> Sum1/1
  Gain/1 -> Sum/1, Sum2/1
  Integrator/1 -> Sum/2
  Gain1/1 -> Integrator/1
  Sum/1 -> req_T/1

== system car/car_model/ice model/local controller/Max speed controller ==
  Enable : EnablePort  StatesWhenEnabling=reset  PropagateVarSize=During execution
  Constant1 : Constant  Value=-T_max
  req_T : Outport  OutputWhenDisabled=reset  InitialOutput=T_max
  wires:
  Constant1/1 -> req_T/1
